simulink model "oog_example"  (R2016a)
settings: Solver=ode5  SolverMode=SingleTasking  StartTime=0.0  StopTime=Ttot  FixedStep=min(Ts_phy,Ts_sim)  RelTol=1e-3
PreLoadFcn:
  | oog_example_init
InitFcn:
  | oog_example_init
values from neighbouring files (symbols this model uses):
  col = {}    [oog_example_init.m]
  flex = {}    [oog_example_init.m]
  systemBase = {}    [oog_example_init.m]
  Ts = Ts_c    (= 0.0001)    [oog_example_init.m]
  Ts_phy = 1*Ts_sim    (= 0.0001)    [oog_example_init.m]
  Ts_sim = 100e-6    (= 0.0001)    [oog_example_init.m]
  wt1 = {}    [oog_example_init.m]
  wt2 = wt1    [oog_example_init.m]
  wt3 = wt1    [oog_example_init.m]
undefined symbols (not defined in the file or in its folder): avr, D1, Delta, DiscIntNeverNeededParam, governor, interface, Lf1, sm
libraries: powerlib x49, simulink_extras x35, pwrsysBasic x30, powerlib_meascontrol x17, pwrsysVICtrl x15, simulink x5, pwrsysVSrc x4, pwrsysTransf x4
(part 2 of 3)

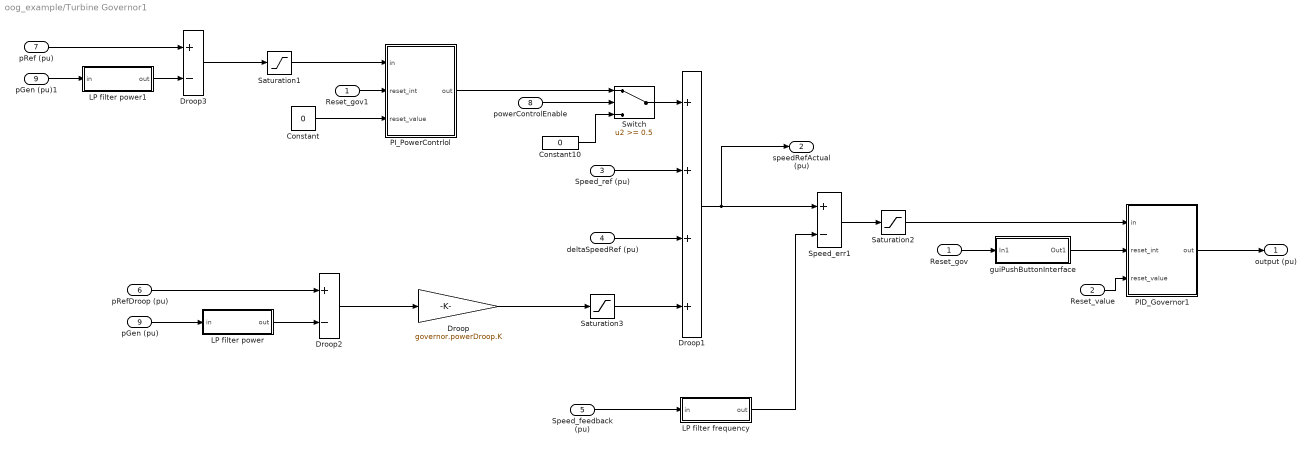
== system oog_example/Turbine Governor1 ==
  Reset_gov : Inport
  Reset_value : Inport  Port=2
  Speed_ref (pu) : Inport  Port=3
  deltaSpeedRef (pu) : Inport  Port=4
  Speed_feedback (pu) : Inport  Port=5
  pRefDroop (pu) : Inport  Port=6
  pRef (pu) : Inport  Port=7
  powerControlEnable : Inport  Port=8
  pGen (pu) : Inport  Port=9
  Constant : Constant  Value=0
  Constant10 : Constant  Value=0  SampleTime=Ts
  Droop : Gain  Gain=governor.powerDroop.K
  Droop1 : Sum  Inputs=++++
  Droop2 : Sum  Inputs=+-
  Droop3 : Sum  Inputs=+-
  LP filter frequency : Subsystem  mask(Discrete first order low pass filter){tau=governor.LPfilterFrequencyMeasurement.T, Ts=Ts, x0=0, y0=0}
      mask prompts: tau "Filter time constant [s]"; Ts "Sampling time [s]"; x0 "Initial input"; y0 "Initial output"
      mask help: Discrete first order low pass filter derived from a continous filter by bilinear transformation.
  LP filter power : Subsystem  mask(Discrete first order low pass filter){tau=governor.LPfilterPowerMeasurementDroop.T, Ts=Ts, x0=0, y0=0}
      mask prompts: tau "Filter time constant [s]"; Ts "Sampling time [s]"; x0 "Initial input"; y0 "Initial output"
      mask help: Discrete first order low pass filter derived from a continous filter by bilinear transformation.
  LP filter power1 : Subsystem  mask(Discrete first order low pass filter){tau=governor.LPfilterPowerMeasurementPowerControl.T, Ts=Ts, x0=0, y0=0}
      mask prompts: tau "Filter time constant [s]"; Ts "Sampling time [s]"; x0 "Initial input"; y0 "Initial output"
      mask help: Discrete first order low pass filter derived from a continous filter by bilinear transformation.
  PID_Governor1 : Subsystem  mask(Discrete PI with parallel form){kp=governor.kP, ki=governor.kI, kd=governor.kd, Tlp=governor.derivativeLP, xi=governor.init, up_sat_limit=governor.saturationUpper, low_sat_limit=governor.saturationLower}
      mask prompts: kp "Proportional gain"; ki "Integral gain"; kd "Derivative gain"; Tlp "Derivative LP filter T"; xi "Initial condition integrator"; up_sat_limit "Saturation upper limit"; low_sat_limit "Saturation lower limit"
      mask help: Discrete PI in parallel form with saturation on the integrator and on the output. The upper and the lower saturation limits are fixed.
  PI_PowerContrlol : Subsystem  mask(Discrete PI with parallel form){kp=governor.powerControl.kP, ki=governor.powerControl.kI, xi=0, up_sat_limit=governor.powerControl.saturationUpper, low_sat_limit=governor.powerControl.saturationLower}
      mask prompts: kp "Proportional gain"; ki "Integral gain"; xi "Initial condition integrator"; up_sat_limit "Saturation upper limit"; low_sat_limit "Saturation lower limit"
      mask help: Discrete PI in parallel form with saturation on the integrator and on the output. The upper and the lower saturation limits are fixed.
  Reset_gov1 : InportShadow
  Saturation1 : Saturate  UpperLimit=governor.powerControl.errMax  LowerLimit=governor.powerControl.errMin
  Saturation2 : Saturate  UpperLimit=governor.speedErrMax  LowerLimit=governor.speedErrMin
  Saturation3 : Saturate  UpperLimit=governor.powerMeasSaturationUpper  LowerLimit=governor.powerMeasSaturationLower
  Speed_err1 : Sum  Inputs=+-
  Switch : Switch  Threshold=0.5
  guiPushButtonInterface : Subsystem
  pGen (pu)1 : InportShadow  Port=9
  output (pu) : Outport
  speedRefActual (pu) : Outport  Port=2
  wires:
  guiPushButtonInterface/1(Out1) -> PID_Governor1/2(reset_int)
  powerControlEnable/1 -> Switch/2
  PI_PowerContrlol/1(out) -> Switch/1
  Constant10/1 -> Switch/3
  Switch/1 -> Droop1/1
  LP filter power1/1(out) -> Droop3/2
  Saturation3/1 -> Droop1/4
  pGen (pu)1/1 -> LP filter power1/1(in)
  Saturation2/1 -> PID_Governor1/1(in)
  deltaSpeedRef (pu)/1 -> Droop1/3
  Constant/1 -> PI_PowerContrlol/3(reset_value)
  Reset_gov1/1 -> PI_PowerContrlol/2(reset_int)
  Saturation1/1 -> PI_PowerContrlol/1(in)
  Droop3/1 -> Saturation1/1
  pRef (pu)/1 -> Droop3/1
  Droop2/1 -> Droop/1
  Reset_value/1 -> PID_Governor1/3(reset_value)
  LP filter power/1(out) -> Droop2/2
  pRefDroop (pu)/1 -> Droop2/1
  pGen (pu)/1 -> LP filter power/1(in)
  Speed_err1/1 -> Saturation2/1
  Droop/1 -> Saturation3/1
  LP filter frequency/1(out) -> Speed_err1/2
  PID_Governor1/1(out) -> output (pu)/1
  Reset_gov/1 -> guiPushButtonInterface/1(In1)
  Droop1/1 -> Speed_err1/1, speedRefActual (pu)/1
  Speed_feedback (pu)/1 -> LP filter frequency/1(in)
  Speed_ref (pu)/1 -> Droop1/2

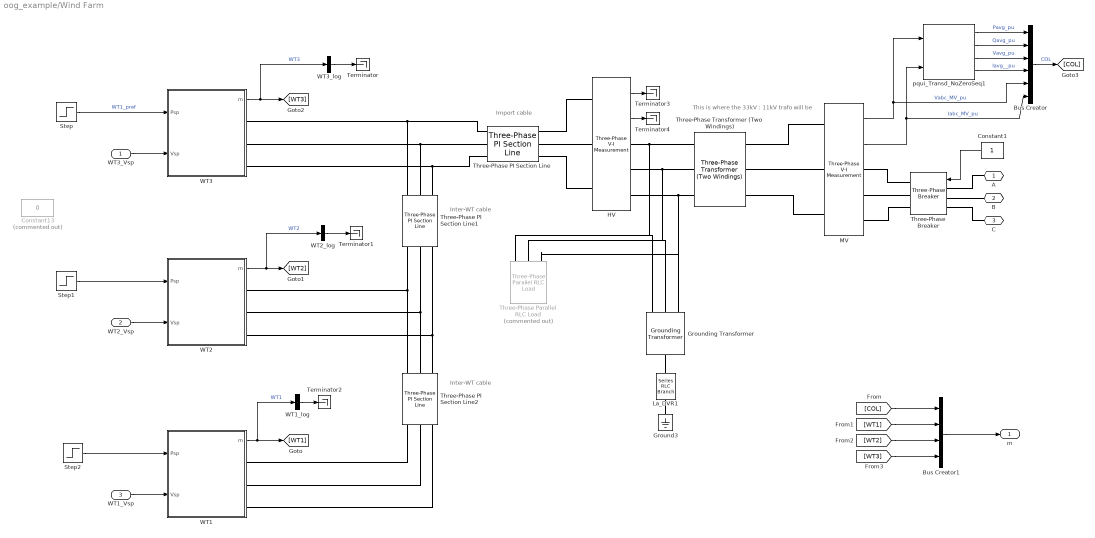
== system oog_example/Wind Farm ==
  note: Import cable
  note: This is where the 33kV : 11kV trafo will be
  note: Inter-WT cable
  note: Inter-WT cable
  WT3_Vsp : Inport
  WT2_Vsp : Inport  Port=2
  WT1_Vsp : Inport  Port=3
  Bus Creator : BusCreator  Inputs=6
  Bus Creator1 : BusCreator  Inputs=4
  Constant1 : Constant  SampleTime=Ts_sim
  Constant13 : Constant  Commented=on  Value=0  SampleTime=Ts_sim
  Ground3 : powerlib/Elements/Ground  LConnTagsString=a
  "Grounding Transformer " : powerlib/Elements/Grounding Transformer   UNITS=pu  NominalPower=[ col.Sn , systemBase.fn ]  NominalVoltage=systemBase.Vn  ZeroSequenceImpedance_pu=[0.025 0.75]  MagnetizationBranch_pu=[500 500]  ZeroSequenceImpedance_SI=[0.052083 589.05]  MagnetizationBranch_SI=[1041.7 3.927e+005]  Measurements=None
  HV : powerlib/Measurements/Three-Phase V-I Measurement  VoltageMeasurement=phase-to-ground  SetLabelV=off  LabelV=vgrid  Vpu=off  VpuLL=off  CurrentMeasurement=yes  SetLabelI=off  LabelI=igrid  Ipu=off  Pbase=sn  Vbase=uab  OutputType=Complex  PhasorSimulation=off  PSBequivalent=0
  La_DVR1 : powerlib/Elements/Series RLC Branch  LConnTagsString=__new0  RConnTagsString=__new0  BranchType=R  Resistance=250  Inductance=Lf1  SetiL0=off  InitialCurrent=0  Capacitance=1.0  Setx0=off  InitialVoltage=0  Measurements=None
  MV : powerlib/Measurements/Three-Phase V-I Measurement  VoltageMeasurement=phase-to-ground  SetLabelV=off  LabelV=vgrid  Vpu=off  VpuLL=off  CurrentMeasurement=yes  SetLabelI=off  LabelI=igrid  Ipu=off  Pbase=sn  Vbase=uab  OutputType=Complex  PhasorSimulation=off  PSBequivalent=0
  Step : Step  Time=6  After=0.73  SampleTime=0
  Step1 : Step  Time=5  After=0.72  SampleTime=0
  Step2 : Step  Time=4  After=0.71  SampleTime=0
  Terminator{,1..4} (5 alike) : Terminator
  Three-Phase PI Section Line : powerlib/Elements/Three-Phase PI Section Line  LConnTagsString=a|b|c  RConnTagsString=A|B|C  Frequency=systemBase.fn  Resistances=[ col.Cable.Rpos col.Cable.Rzero]  Inductances=[ col.Cable.Lpos col.Cable.Lzero]  Capacitances=[col.Cable.Cpos col.Cable.Czero]  Length=col.Cable.Limport
  Three-Phase PI Section Line1 : powerlib/Elements/Three-Phase PI Section Line  LConnTagsString=a|b|c  RConnTagsString=A|B|C  Frequency=systemBase.fn  Resistances=[ col.Cable.Rpos col.Cable.Rzero]  Inductances=[ col.Cable.Lpos col.Cable.Lzero]  Capacitances=[col.Cable.Cpos col.Cable.Czero]  Length=col.Cable.LinterWT
  Three-Phase PI Section Line2 : powerlib/Elements/Three-Phase PI Section Line  LConnTagsString=a|b|c  RConnTagsString=A|B|C  Frequency=systemBase.fn  Resistances=[ col.Cable.Rpos col.Cable.Rzero]  Inductances=[ col.Cable.Lpos col.Cable.Lzero]  Capacitances=[col.Cable.Cpos col.Cable.Czero]  Length=col.Cable.LinterWT
  Three-Phase Parallel RLC Load : powerlib/Elements/Three-Phase Parallel RLC Load  Commented=on  LConnTagsString=A|B|C  Configuration=Y (grounded)  NominalVoltage=col.Un  Vabc=[1e3 1e3 1e3]  Vabcp=[1e3 1e3 1e3]  NominalFrequency=systemBase.fn  UnbalancedPower=off  ActivePower=100  InductivePower=0  CapacitivePower=0  Pabc=[10e3 9e3 11e3]  QLabc=[100 90 110]  QCabc=[100 90 110]  Pabcp=[10e3 9e3 11e3]  QLabcp=[100 90 110]  QCabcp=[100 90 110]  Measurements=None  LoadType=constant Z
  Three-Phase Transformer (Two Windings) : powerlib/Elements/Three-Phase Transformer (Two Windings)  Winding1Connection=Y  Winding2Connection=Delta (D1)  CoreType=Three-limb core (core-type)  SetSaturation=off  Hysteresis=off  DataFile='hysteresis'  SetInitialFlux=off  Measurements=None  UNITS=pu  NominalPower=[ col.Sn , systemBase.fn ]  Winding1=[ systemBase.Vn , col.Trafo.rsc/2 , col.Trafo.xsc/2 ]  Winding2=[ col.Un , col.Trafo.rsc/2 , col.Trafo.xsc/2 ]  Rm=500  Lm=500  L0=0.5  Saturation=[ 0,0 ; 0.0024,1.2 ; 1.0,1.52 ]  InitialFluxes=[0 0 0]  MoreParameters=off  BreakLoop=off  DataType=off  TransfoNumber=1
  Three-Phase Breaker : powerlib/Elements/Three-Phase Breaker  InitialState=closed  SwitchA=on  SwitchB=on  SwitchC=on  SwitchTimes="[1/60  5/60]"  External=on  BreakerResistance=0.01  SnubberResistance=1e6  SnubberCapacitance=1e9  Measurements=None
  WT1 : Subsystem
  WT1_log : BusSelector  OutputSignals=Pavg_pu,Qavg_pu,Vavg_pu,Vdc_pu,Idc_pu  OutputAsBus=on
  WT2 : Subsystem
  WT2_log : BusSelector  OutputSignals=Pavg_pu,Qavg_pu,Vavg_pu,Vdc_pu,Idc_pu  OutputAsBus=on
  WT3 : Subsystem
  WT3_log : BusSelector  OutputSignals=Pavg_pu,Qavg_pu,Vavg_pu,Vdc_pu,Idc_pu  OutputAsBus=on
  pqui_Transd_NoZeroSeq1 : pwrsysBasic/pqui_Transd_NoZeroSeq  Sn=col.Sn  Uanp=systemBase.Vn_phase*sqrt(2)  Iap=col.Iap*(col.Un/systemBase.Vn_phase)
  A : PMIOPort  Port=1  Side=Right
  B : PMIOPort  Port=2  Side=Right
  C : PMIOPort  Port=3  Side=Right
  m : Outport
  wires:
  Constant1/1 -> Three-Phase Breaker/1
  MV/1 -> Bus Creator/5, pqui_Transd_NoZeroSeq1/1  "Vabc_MV_pu"
  HV/1 -> Terminator3/1
  HV/2 -> Terminator4/1
  MV/2 -> pqui_Transd_NoZeroSeq1/2, Bus Creator/6  "Iabc_MV_pu"
  pqui_Transd_NoZeroSeq1/1 -> Bus Creator/1  "Pavg_pu"
  pqui_Transd_NoZeroSeq1/4 -> Bus Creator/4  "Iavg__pu"
  pqui_Transd_NoZeroSeq1/2 -> Bus Creator/2  "Qavg_pu"
  pqui_Transd_NoZeroSeq1/3 -> Bus Creator/3  "Vavg_pu"
  Bus Creator/1 -> [COL]  "COL"
  WT3/1(m) -> WT3_log/1, [WT3]  "WT3"
  WT2/1(m) -> WT2_log/1, [WT2]  "WT2"
  WT3_Vsp/1 -> WT3/2(Vsp)
  WT2_Vsp/1 -> WT2/2(Vsp)
  WT1_Vsp/1 -> WT1/2(Vsp)
  Bus Creator1/1 -> m/1
  [COL] -> Bus Creator1/1
  [WT1] -> Bus Creator1/2
  [WT2] -> Bus Creator1/3
  [WT3] -> Bus Creator1/4
  WT3_log/1 -> Terminator/1
  WT2_log/1 -> Terminator1/1
  WT1/1(m) -> WT1_log/1, [WT1]  "WT1"
  WT1_log/1 -> Terminator2/1
  Step/1 -> WT3/1(Psp)  "WT1_pref"
  Step1/1 -> WT2/1(Psp)
  Step2/1 -> WT1/1(Psp)
  connections:
  Three-Phase Breaker/RConn3 -- MV/RConn3
  Three-Phase Transformer (Two Windings)/LConn3 -- MV/LConn3
  Three-Phase Transformer (Two Windings)/LConn1 -- MV/LConn1
  Three-Phase Transformer (Two Windings)/LConn2 -- MV/LConn2
  MV/RConn1 -- Three-Phase Breaker/RConn1
  Three-Phase PI Section Line/RConn2 -- HV/LConn2
  Three-Phase Breaker/RConn2 -- MV/RConn2
  HV/LConn1 -- Three-Phase PI Section Line/RConn1
  HV/LConn3 -- Three-Phase PI Section Line/RConn3
  Three-Phase Breaker/LConn2 -- B/RConn1
  Three-Phase PI Section Line1/LConn3 -- WT3/RConn3 -- Three-Phase PI Section Line/LConn3
  Three-Phase Breaker/LConn1 -- A/RConn1
  Three-Phase Breaker/LConn3 -- C/RConn1
  Three-Phase PI Section Line1/LConn2 -- WT3/RConn2 -- Three-Phase PI Section Line/LConn2
  Three-Phase PI Section Line/LConn1 -- WT3/RConn1 -- Three-Phase PI Section Line1/LConn1
  Three-Phase PI Section Line2/LConn1 -- WT2/RConn1 -- Three-Phase PI Section Line1/RConn1
  Three-Phase PI Section Line2/LConn2 -- WT2/RConn2 -- Three-Phase PI Section Line1/RConn2
  Three-Phase PI Section Line2/LConn3 -- WT2/RConn3 -- Three-Phase PI Section Line1/RConn3
  WT1/RConn1 -- Three-Phase PI Section Line2/RConn1
  WT1/RConn2 -- Three-Phase PI Section Line2/RConn2
  WT1/RConn3 -- Three-Phase PI Section Line2/RConn3
  HV/RConn1 -- Three-Phase Parallel RLC Load/LConn1 -- "Grounding Transformer "/LConn3 -- Three-Phase Transformer (Two Windings)/RConn1
  HV/RConn2 -- Three-Phase Parallel RLC Load/LConn2 -- "Grounding Transformer "/LConn2 -- Three-Phase Transformer (Two Windings)/RConn2
  HV/RConn3 -- Three-Phase Parallel RLC Load/LConn3 -- "Grounding Transformer "/LConn1 -- Three-Phase Transformer (Two Windings)/RConn3
  La_DVR1/RConn1 -- "Grounding Transformer "/RConn1
  La_DVR1/LConn1 -- Ground3/LConn1

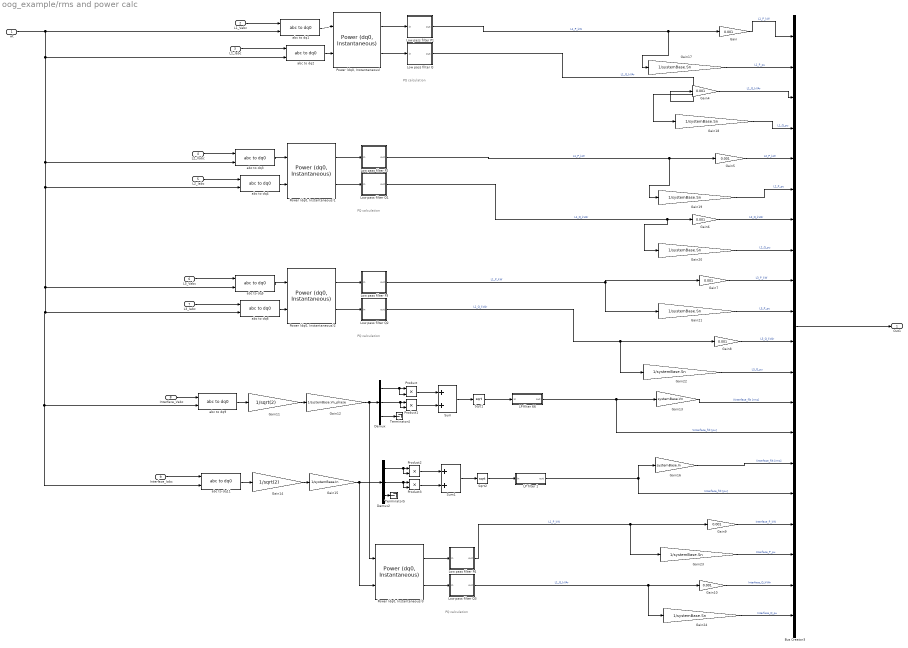
== system oog_example/rms and power calc ==
  note: PQ calculation
  note: PQ calculation
  note: PQ calculation
  note: PQ calculation
  wt : Inport
  L1_Vabc : Inport  Port=2
  L1_Iabc : Inport  Port=3
  L2_Vabc : Inport  Port=4
  L2_Iabc : Inport  Port=5
  L3_Vabc : Inport  Port=6
  L3_Iabc : Inport  Port=7
  Interface_Vabc : Inport  Port=8
  Interface_Iabc : Inport  Port=9
  Bus Creator3 : BusCreator  Inputs=20
  Demux : Demux  Outputs=3
  Demux2 : Demux  Outputs=3
  Gain{,4..10} (8 alike) : Gain  Gain=0.001
  Gain11 : Gain  Gain=1/sqrt(2)
  Gain12 : Gain  Gain=1/systemBase.Vn_phase
  Gain13 : Gain  Gain=systemBase.Vn
  Gain14 : Gain  Gain=1/sqrt(2)
  Gain15 : Gain  Gain=1/systemBase.In
  Gain16 : Gain  Gain=systemBase.In
  Gain{17..24} (8 alike) : Gain  Gain=1/systemBase.Sn
  LP filter 1 : Subsystem  mask(Discrete first order low pass filter){tau=sm.V_measure_T, Ts=Ts, x0=avr.init, y0=avr.init}
      mask prompts: tau "Filter time constant [s]"; Ts "Sampling time [s]"; x0 "Initial input"; y0 "Initial output"
      mask help: Discrete first order low pass filter derived from a continous filter by bilinear transformation.
  LP filter 66 : Subsystem  mask(Discrete first order low pass filter){tau=sm.V_measure_T, Ts=Ts, x0=avr.init, y0=avr.init}
      mask prompts: tau "Filter time constant [s]"; Ts "Sampling time [s]"; x0 "Initial input"; y0 "Initial output"
      mask help: Discrete first order low pass filter derived from a continous filter by bilinear transformation.
  Low pass filter P1 : Subsystem  mask(Discrete first order low pass filter){tau=sm.P_measure, Ts=Ts, x0=0, y0=0}
      mask prompts: tau "Filter time constant [s]"; Ts "Sampling time [s]"; x0 "Initial input"; y0 "Initial output"
      mask help: Discrete first order low pass filter derived from a continous filter by bilinear transformation.
  Low pass filter P2 : Subsystem  mask(Discrete first order low pass filter){tau=sm.P_measure, Ts=Ts, x0=0, y0=0}
      mask prompts: tau "Filter time constant [s]"; Ts "Sampling time [s]"; x0 "Initial input"; y0 "Initial output"
      mask help: Discrete first order low pass filter derived from a continous filter by bilinear transformation.
  Low pass filter P3 : Subsystem  mask(Discrete first order low pass filter){tau=sm.P_measure, Ts=Ts, x0=0, y0=0}
      mask prompts: tau "Filter time constant [s]"; Ts "Sampling time [s]"; x0 "Initial input"; y0 "Initial output"
      mask help: Discrete first order low pass filter derived from a continous filter by bilinear transformation.
  Low pass filter P4 : Subsystem  mask(Discrete first order low pass filter){tau=sm.P_measure, Ts=Ts, x0=0, y0=0}
      mask prompts: tau "Filter time constant [s]"; Ts "Sampling time [s]"; x0 "Initial input"; y0 "Initial output"
      mask help: Discrete first order low pass filter derived from a continous filter by bilinear transformation.
  Low pass filter Q : Subsystem  mask(Discrete first order low pass filter){tau=sm.Q_measure, Ts=Ts, x0=0, y0=0}
      mask prompts: tau "Filter time constant [s]"; Ts "Sampling time [s]"; x0 "Initial input"; y0 "Initial output"
      mask help: Discrete first order low pass filter derived from a continous filter by bilinear transformation.
  Low pass filter Q1 : Subsystem  mask(Discrete first order low pass filter){tau=sm.Q_measure, Ts=Ts, x0=0, y0=0}
      mask prompts: tau "Filter time constant [s]"; Ts "Sampling time [s]"; x0 "Initial input"; y0 "Initial output"
      mask help: Discrete first order low pass filter derived from a continous filter by bilinear transformation.
  Low pass filter Q2 : Subsystem  mask(Discrete first order low pass filter){tau=sm.Q_measure, Ts=Ts, x0=0, y0=0}
      mask prompts: tau "Filter time constant [s]"; Ts "Sampling time [s]"; x0 "Initial input"; y0 "Initial output"
      mask help: Discrete first order low pass filter derived from a continous filter by bilinear transformation.
  Low pass filter Q3 : Subsystem  mask(Discrete first order low pass filter){tau=sm.Q_measure, Ts=Ts, x0=0, y0=0}
      mask prompts: tau "Filter time constant [s]"; Ts "Sampling time [s]"; x0 "Initial input"; y0 "Initial output"
      mask help: Discrete first order low pass filter derived from a continous filter by bilinear transformation.
  Power (dq0, Instantaneous){,1..3} (4 alike) : powerlib_meascontrol/Measurements/Power (dq0, Instantaneous)
  Product{,1..3} (4 alike) : Product
  Sqrt1 : Sqrt  SaturateOnIntegerOverflow=on
  Sqrt2 : Sqrt  SaturateOnIntegerOverflow=on
  Sum : Sum
  Sum1 : Sum
  Terminator4 : Terminator
  Terminator5 : Terminator
  abc to dq{1..6,9,11} (8 alike) : powerlib_meascontrol/Transformations/abc to dq0  Alignment=Aligned with phase A axis
  Out1 : Outport
  wires:
  "Power (dq0, Instantaneous)"/1 -> Low pass filter P1/1(in)
  Gain22/1 -> Bus Creator3/12  "L3_Q_pu"
  Gain24/1 -> Bus Creator3/20  "Interface_Q_pu"
  Gain19/1 -> Bus Creator3/6  "L2_P_pu"
  Gain5/1 -> Bus Creator3/5  "L2_P_kW"
  Gain18/1 -> Bus Creator3/4  "L1_Q_pu"
  Gain4/1 -> Bus Creator3/3  "L1_Q_kVAr"
  Gain17/1 -> Bus Creator3/2  "L1_P_pu"
  wt/1 -> abc to dq1/2, abc to dq2/2, abc to dq3/2, abc to dq4/2, abc to dq5/2, abc to dq9/2, abc to dq11/2, abc to dq6/2
  Interface_Iabc/1 -> abc to dq11/1
  abc to dq11/1 -> Gain14/1
  Gain21/1 -> Bus Creator3/10  "L3_P_pu"
  Sqrt2/1 -> LP filter 1/1(in)
  Gain23/1 -> Bus Creator3/18  "Interface_P_pu"
  Gain20/1 -> Bus Creator3/8  "L2_Q_pu"
  Gain10/1 -> Bus Creator3/19  "Interface_Q_kVAr"
  "Power (dq0, Instantaneous)3"/2 -> Low pass filter Q3/1(in)
  LP filter 1/1(out) -> Gain16/1, Bus Creator3/16  "Iinterface_filt [pu]"
  Interface_Vabc/1 -> abc to dq9/1
  Low pass filter Q2/1(out) -> Gain22/1, Gain8/1  "L1_Q_kVAr"
  "Power (dq0, Instantaneous)3"/1 -> Low pass filter P4/1(in)
  Low pass filter P3/1(out) -> Gain7/1, Gain21/1  "L1_P_kW"
  abc to dq9/1 -> Gain11/1
  Low pass filter P4/1(out) -> Gain9/1, Gain23/1  "L1_P_kW"
  Gain16/1 -> Bus Creator3/15  "Iinterfase_filt [rms]"
  Product2/1 -> Sum1/1
  Demux2/1 -> Product2/1, Product2/2
  LP filter 66/1(out) -> Bus Creator3/14, Gain13/1  "Vinterface_filt [pu]"
  Product/1 -> Sum/1
  Gain11/1 -> Gain12/1
  Gain9/1 -> Bus Creator3/17  "Interface_P_kW"
  Sum/1 -> Sqrt1/1
  Gain15/1 -> Demux2/1, "Power (dq0, Instantaneous)3"/2
  Gain12/1 -> Demux/1, "Power (dq0, Instantaneous)3"/1
  Product3/1 -> Sum1/2
  Product1/1 -> Sum/2
  Demux/1 -> Product/1, Product/2
  Low pass filter Q3/1(out) -> Gain24/1, Gain10/1  "L1_Q_kVAr"
  Sqrt1/1 -> LP filter 66/1(in)
  Gain14/1 -> Gain15/1
  Demux2/2 -> Product3/1, Product3/2
  Gain13/1 -> Bus Creator3/13  "Vinterfase_filt [rms]"
  Sum1/1 -> Sqrt2/1
  Demux/2 -> Product1/1, Product1/2
  "Power (dq0, Instantaneous)1"/1 -> Low pass filter P2/1(in)
  Gain8/1 -> Bus Creator3/11  "L3_Q_kVAr"
  L3_Vabc/1 -> abc to dq5/1
  L2_Iabc/1 -> abc to dq4/1
  L2_Vabc/1 -> abc to dq3/1
  abc to dq3/1 -> "Power (dq0, Instantaneous)1"/1
  Gain7/1 -> Bus Creator3/9  "L3_P_kW"
  L3_Iabc/1 -> abc to dq6/1
  "Power (dq0, Instantaneous)2"/1 -> Low pass filter P3/1(in)
  Low pass filter Q/1(out) -> Gain4/1, Gain18/1  "L1_Q_kVAr"
  "Power (dq0, Instantaneous)1"/2 -> Low pass filter Q1/1(in)
  "Power (dq0, Instantaneous)2"/2 -> Low pass filter Q2/1(in)
  abc to dq4/1 -> "Power (dq0, Instantaneous)1"/2
  Low pass filter P1/1(out) -> Gain/1, Gain17/1  "L1_P_kW"
  abc to dq5/1 -> "Power (dq0, Instantaneous)2"/1
  Low pass filter Q1/1(out) -> Gain6/1, Gain20/1  "L1_Q_kVAr"
  Bus Creator3/1 -> Out1/1
  abc to dq6/1 -> "Power (dq0, Instantaneous)2"/2
  Low pass filter P2/1(out) -> Gain5/1, Gain19/1  "L1_P_kW"
  Gain6/1 -> Bus Creator3/7  "L2_Q_kVAr"
  L1_Iabc/1 -> abc to dq2/1
  L1_Vabc/1 -> abc to dq1/1
  abc to dq2/1 -> "Power (dq0, Instantaneous)"/2
  abc to dq1/1 -> "Power (dq0, Instantaneous)"/1
  Gain/1 -> Bus Creator3/1  "L1_P_kW"
  "Power (dq0, Instantaneous)"/2 -> Low pass filter Q/1(in)
  Demux2/3 -> Terminator5/1
  Demux/3 -> Terminator4/1

== system oog_example/Automatic voltage regulator/LP filter active power ==
  in : Inport
  Discrete Transfer Fcn (with initial outputs) : simulink_extras/Additional Discrete/Discrete Transfer Fcn (with initial outputs)  N=[1/tau*Ts/2 1/tau*Ts/2]  D=[(1/tau*Ts/2+1) (1/tau*Ts/2-1)]  U0=x0  Y0=y0  TS=Ts
  out : Outport
  wires:
  in/1 -> Discrete Transfer Fcn (with initial outputs)/1
  Discrete Transfer Fcn (with initial outputs)/1 -> out/1

== system oog_example/Automatic voltage regulator/LP filter frequency ==
  in : Inport
  Discrete Transfer Fcn (with initial outputs) : simulink_extras/Additional Discrete/Discrete Transfer Fcn (with initial outputs)  N=[1/tau*Ts/2 1/tau*Ts/2]  D=[(1/tau*Ts/2+1) (1/tau*Ts/2-1)]  U0=x0  Y0=y0  TS=Ts
  out : Outport
  wires:
  Discrete Transfer Fcn (with initial outputs)/1 -> out/1
  in/1 -> Discrete Transfer Fcn (with initial outputs)/1

== system oog_example/Automatic voltage regulator/LP filter frequency1 ==
  in : Inport
  Discrete Transfer Fcn (with initial outputs) : simulink_extras/Additional Discrete/Discrete Transfer Fcn (with initial outputs)  N=[1/tau*Ts/2 1/tau*Ts/2]  D=[(1/tau*Ts/2+1) (1/tau*Ts/2-1)]  U0=x0  Y0=y0  TS=Ts
  out : Outport
  wires:
  Discrete Transfer Fcn (with initial outputs)/1 -> out/1
  in/1 -> Discrete Transfer Fcn (with initial outputs)/1

== system oog_example/Automatic voltage regulator/LP filter reactive power ==
  in : Inport
  Discrete Transfer Fcn (with initial outputs) : simulink_extras/Additional Discrete/Discrete Transfer Fcn (with initial outputs)  N=[1/tau*Ts/2 1/tau*Ts/2]  D=[(1/tau*Ts/2+1) (1/tau*Ts/2-1)]  U0=x0  Y0=y0  TS=Ts
  out : Outport
  wires:
  Discrete Transfer Fcn (with initial outputs)/1 -> out/1
  in/1 -> Discrete Transfer Fcn (with initial outputs)/1

== system oog_example/Automatic voltage regulator/PID_Governor1 ==
  in : Inport
  reset_int : Inport  Port=2
  reset_value : Inport  Port=3
  Discrete Derivative : simulink/Discrete/Discrete Derivative  gainval=1.0  ICPrevScaledInput=0.0  InputProcessing=Inherited  OutMin=[]  OutMax=[]  OutDataType=fixdt(1, 16)  OutScaling=2^-10  DoSatur=off
  Discrete-Time Integrator : DiscreteIntegrator  IntegratorMethod=Integration: Trapezoidal  ExternalReset=level  InitialConditionSource=external  InitialCondition=xi  InitialConditionSetting=State (most efficient)  SampleTime=Ts  LimitOutput=on  UpperSaturationLimit=up_sat_limit  LowerSaturationLimit=low_sat_limit  ICPrevOutput=DiscIntNeverNeededParam  ICPrevScaledInput=DiscIntNeverNeededParam
  Integral Gain : Gain  DisableCoverage=on  Gain=ki
  Integral Gain1 : Gain  DisableCoverage=on  Gain=kd
  LP filter power : Subsystem  mask(Discrete first order low pass filter){tau=governor.derivativeLP, Ts=Ts, x0=0, y0=0}
      mask prompts: tau "Filter time constant [s]"; Ts "Sampling time [s]"; x0 "Initial input"; y0 "Initial output"
      mask help: Discrete first order low pass filter derived from a continous filter by bilinear transformation.
  P+I : Sum  Inputs=+++
  Proportional Gain : Gain  DisableCoverage=on  Gain=kp
  Saturation : Saturate  UpperLimit=up_sat_limit  LowerLimit=low_sat_limit
  out : Outport
  wires:
  LP filter power/1(out) -> Discrete Derivative/1
  Discrete Derivative/1 -> P+I/3
  Integral Gain1/1 -> LP filter power/1(in)
  reset_value/1 -> Discrete-Time Integrator/3
  reset_int/1 -> Discrete-Time Integrator/2
  Saturation/1 -> out/1
  Proportional Gain/1 -> P+I/1
  in/1 -> Integral Gain/1, Integral Gain1/1, Proportional Gain/1
  P+I/1 -> Saturation/1
  Integral Gain/1 -> Discrete-Time Integrator/1
  Discrete-Time Integrator/1 -> P+I/2

== system oog_example/Automatic voltage regulator/guiPushButtonInterface ==
  In1 : Inport
  Data Type Conversion6 : DataTypeConversion  OutDataTypeStr=double  RndMeth=Round
  Detect Change : simulink/Logic and Bit Operations/Detect Change  vinit=0  InputProcessing=Inherited  OutDataTypeStr=boolean
  IC1 : InitialCondition  Value=0
  Out1 : Outport
  wires:
  IC1/1 -> Out1/1
  Data Type Conversion6/1 -> IC1/1
  Detect Change/1 -> Data Type Conversion6/1
  In1/1 -> Detect Change/1

== system oog_example/Rotation1/guiPushButtonInterface ==
  In1 : Inport
  Data Type Conversion6 : DataTypeConversion  OutDataTypeStr=double  RndMeth=Round
  Detect Change : simulink/Logic and Bit Operations/Detect Change  vinit=0  InputProcessing=Inherited  OutDataTypeStr=boolean
  IC1 : InitialCondition  Value=0
  Out1 : Outport
  wires:
  IC1/1 -> Out1/1
  Data Type Conversion6/1 -> IC1/1
  Detect Change/1 -> Data Type Conversion6/1
  In1/1 -> Detect Change/1

== system oog_example/SM_simple/LP filter  ==
  in : Inport
  Discrete Transfer Fcn (with initial outputs) : simulink_extras/Additional Discrete/Discrete Transfer Fcn (with initial outputs)  N=[1/tau*Ts/2 1/tau*Ts/2]  D=[(1/tau*Ts/2+1) (1/tau*Ts/2-1)]  U0=x0  Y0=y0  TS=Ts
  out : Outport
  wires:
  Discrete Transfer Fcn (with initial outputs)/1 -> out/1
  in/1 -> Discrete Transfer Fcn (with initial outputs)/1

== system oog_example/SM_simple/LP filter 1 ==
  in : Inport
  Discrete Transfer Fcn (with initial outputs) : simulink_extras/Additional Discrete/Discrete Transfer Fcn (with initial outputs)  N=[1/tau*Ts/2 1/tau*Ts/2]  D=[(1/tau*Ts/2+1) (1/tau*Ts/2-1)]  U0=x0  Y0=y0  TS=Ts
  out : Outport
  wires:
  Discrete Transfer Fcn (with initial outputs)/1 -> out/1
  in/1 -> Discrete Transfer Fcn (with initial outputs)/1

== system oog_example/SM_simple/LP filter 2 ==
  in : Inport
  Discrete Transfer Fcn (with initial outputs) : simulink_extras/Additional Discrete/Discrete Transfer Fcn (with initial outputs)  N=[1/tau*Ts/2 1/tau*Ts/2]  D=[(1/tau*Ts/2+1) (1/tau*Ts/2-1)]  U0=x0  Y0=y0  TS=Ts
  out : Outport
  wires:
  in/1 -> Discrete Transfer Fcn (with initial outputs)/1
  Discrete Transfer Fcn (with initial outputs)/1 -> out/1

== system oog_example/SM_simple/LP filter 3 ==
  in : Inport
  Discrete Transfer Fcn (with initial outputs) : simulink_extras/Additional Discrete/Discrete Transfer Fcn (with initial outputs)  N=[1/tau*Ts/2 1/tau*Ts/2]  D=[(1/tau*Ts/2+1) (1/tau*Ts/2-1)]  U0=x0  Y0=y0  TS=Ts
  out : Outport
  wires:
  in/1 -> Discrete Transfer Fcn (with initial outputs)/1
  Discrete Transfer Fcn (with initial outputs)/1 -> out/1

== system oog_example/SM_simple/LP filter 3  ==
  in : Inport
  Discrete Transfer Fcn (with initial outputs) : simulink_extras/Additional Discrete/Discrete Transfer Fcn (with initial outputs)  N=[1/tau*Ts/2 1/tau*Ts/2]  D=[(1/tau*Ts/2+1) (1/tau*Ts/2-1)]  U0=x0  Y0=y0  TS=Ts
  out : Outport
  wires:
  Discrete Transfer Fcn (with initial outputs)/1 -> out/1
  in/1 -> Discrete Transfer Fcn (with initial outputs)/1

== system oog_example/SM_simple/LP filter 3 1 ==
  in : Inport
  Discrete Transfer Fcn (with initial outputs) : simulink_extras/Additional Discrete/Discrete Transfer Fcn (with initial outputs)  N=[1/tau*Ts/2 1/tau*Ts/2]  D=[(1/tau*Ts/2+1) (1/tau*Ts/2-1)]  U0=x0  Y0=y0  TS=Ts
  out : Outport
  wires:
  Discrete Transfer Fcn (with initial outputs)/1 -> out/1
  in/1 -> Discrete Transfer Fcn (with initial outputs)/1

== system oog_example/SM_simple/LP filter 3 2 ==
  in : Inport
  Discrete Transfer Fcn (with initial outputs) : simulink_extras/Additional Discrete/Discrete Transfer Fcn (with initial outputs)  N=[1/tau*Ts/2 1/tau*Ts/2]  D=[(1/tau*Ts/2+1) (1/tau*Ts/2-1)]  U0=x0  Y0=y0  TS=Ts
  out : Outport
  wires:
  Discrete Transfer Fcn (with initial outputs)/1 -> out/1
  in/1 -> Discrete Transfer Fcn (with initial outputs)/1

== system oog_example/SM_simple/LP filter 4 ==
  in : Inport
  Discrete Transfer Fcn (with initial outputs) : simulink_extras/Additional Discrete/Discrete Transfer Fcn (with initial outputs)  N=[1/tau*Ts/2 1/tau*Ts/2]  D=[(1/tau*Ts/2+1) (1/tau*Ts/2-1)]  U0=x0  Y0=y0  TS=Ts
  out : Outport
  wires:
  Discrete Transfer Fcn (with initial outputs)/1 -> out/1
  in/1 -> Discrete Transfer Fcn (with initial outputs)/1

== system oog_example/SM_simple/LP filter 5 ==
  in : Inport
  Discrete Transfer Fcn (with initial outputs) : simulink_extras/Additional Discrete/Discrete Transfer Fcn (with initial outputs)  N=[1/tau*Ts/2 1/tau*Ts/2]  D=[(1/tau*Ts/2+1) (1/tau*Ts/2-1)]  U0=x0  Y0=y0  TS=Ts
  out : Outport
  wires:
  Discrete Transfer Fcn (with initial outputs)/1 -> out/1
  in/1 -> Discrete Transfer Fcn (with initial outputs)/1

== system oog_example/SM_simple/LP filter 6 ==
  in : Inport
  Discrete Transfer Fcn (with initial outputs) : simulink_extras/Additional Discrete/Discrete Transfer Fcn (with initial outputs)  N=[1/tau*Ts/2 1/tau*Ts/2]  D=[(1/tau*Ts/2+1) (1/tau*Ts/2-1)]  U0=x0  Y0=y0  TS=Ts
  out : Outport
  wires:
  in/1 -> Discrete Transfer Fcn (with initial outputs)/1
  Discrete Transfer Fcn (with initial outputs)/1 -> out/1

== system oog_example/SM_simple/LP filter 66 ==
  in : Inport
  Discrete Transfer Fcn (with initial outputs) : simulink_extras/Additional Discrete/Discrete Transfer Fcn (with initial outputs)  N=[1/tau*Ts/2 1/tau*Ts/2]  D=[(1/tau*Ts/2+1) (1/tau*Ts/2-1)]  U0=x0  Y0=y0  TS=Ts
  out : Outport
  wires:
  Discrete Transfer Fcn (with initial outputs)/1 -> out/1
  in/1 -> Discrete Transfer Fcn (with initial outputs)/1

== system oog_example/SM_simple/LP filter 67 ==
  in : Inport
  Discrete Transfer Fcn (with initial outputs) : simulink_extras/Additional Discrete/Discrete Transfer Fcn (with initial outputs)  N=[1/tau*Ts/2 1/tau*Ts/2]  D=[(1/tau*Ts/2+1) (1/tau*Ts/2-1)]  U0=x0  Y0=y0  TS=Ts
  out : Outport
  wires:
  Discrete Transfer Fcn (with initial outputs)/1 -> out/1
  in/1 -> Discrete Transfer Fcn (with initial outputs)/1

== system oog_example/SM_simple/Low pass filter P1 ==
  in : Inport
  Discrete Transfer Fcn (with initial outputs) : simulink_extras/Additional Discrete/Discrete Transfer Fcn (with initial outputs)  N=[1/tau*Ts/2 1/tau*Ts/2]  D=[(1/tau*Ts/2+1) (1/tau*Ts/2-1)]  U0=x0  Y0=y0  TS=Ts
  out : Outport
  wires:
  Discrete Transfer Fcn (with initial outputs)/1 -> out/1
  in/1 -> Discrete Transfer Fcn (with initial outputs)/1

== system oog_example/SM_simple/Low pass filter Q ==
  in : Inport
  Discrete Transfer Fcn (with initial outputs) : simulink_extras/Additional Discrete/Discrete Transfer Fcn (with initial outputs)  N=[1/tau*Ts/2 1/tau*Ts/2]  D=[(1/tau*Ts/2+1) (1/tau*Ts/2-1)]  U0=x0  Y0=y0  TS=Ts
  out : Outport
  wires:
  Discrete Transfer Fcn (with initial outputs)/1 -> out/1
  in/1 -> Discrete Transfer Fcn (with initial outputs)/1

== system oog_example/SM_simple/powerCalcAndFilt1 ==
  note: Low pass filter power measurement
  Vabc : Inport
  Iabc : Inport  Port=2
  LP filter frequency1 : Subsystem  mask(Discrete first order low pass filter){tau=sm.P_measure, Ts=Ts, x0=avr.init, y0=avr.init}
      mask prompts: tau "Filter time constant [s]"; Ts "Sampling time [s]"; x0 "Initial input"; y0 "Initial output"
      mask help: Discrete first order low pass filter derived from a continous filter by bilinear transformation.
  LP filter frequency2 : Subsystem  mask(Discrete first order low pass filter){tau=sm.Q_measure, Ts=Ts, x0=avr.init, y0=avr.init}
      mask prompts: tau "Filter time constant [s]"; Ts "Sampling time [s]"; x0 "Initial input"; y0 "Initial output"
      mask help: Discrete first order low pass filter derived from a continous filter by bilinear transformation.
  "Power (3ph, Instantaneous)1" : powerlib_meascontrol/Measurements/Power (3ph, Instantaneous)
  P_filt : Outport
  Q_filt1 : Outport  Port=2
  wires:
  LP filter frequency2/1(out) -> Q_filt1/1
  LP filter frequency1/1(out) -> P_filt/1
  "Power (3ph, Instantaneous)1"/2 -> LP filter frequency2/1(in)
  Iabc/1 -> "Power (3ph, Instantaneous)1"/2
  Vabc/1 -> "Power (3ph, Instantaneous)1"/1
  "Power (3ph, Instantaneous)1"/1 -> LP filter frequency1/1(in)

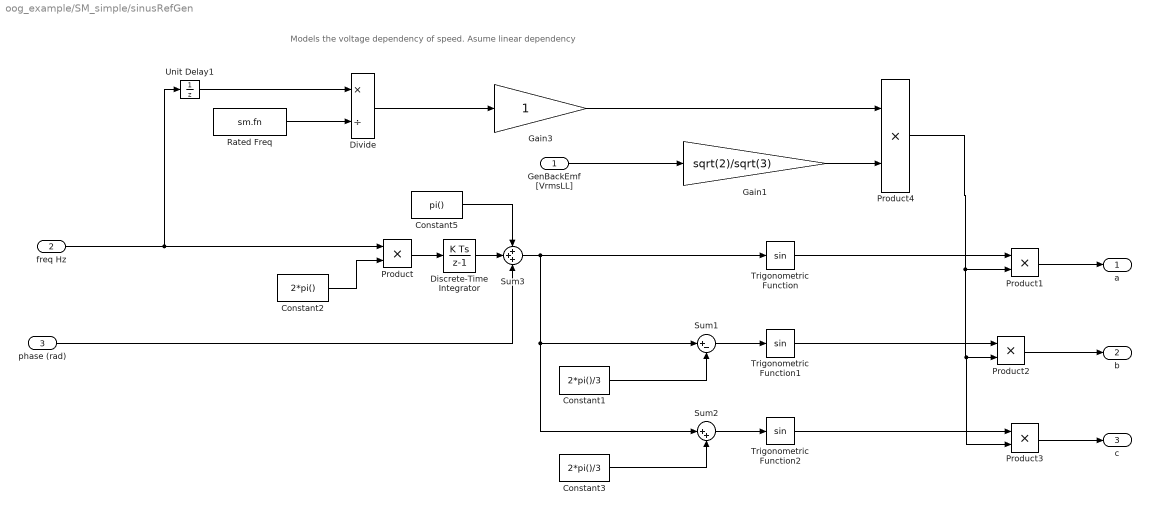
== system oog_example/SM_simple/sinusRefGen ==
  note: Models the voltage dependency of speed. Asume linear dependency
  GenBackEmf [VrmsLL] : Inport
  freq Hz : Inport  Port=2
  phase (rad) : Inport  Port=3
  Constant1 : Constant  Value=2*pi()/3  SampleTime=-1
  Constant2 : Constant  Value=2*pi()  SampleTime=-1
  Constant3 : Constant  Value=2*pi()/3  SampleTime=-1
  Constant5 : Constant  Value=pi()  SampleTime=-1
  Discrete-Time Integrator : DiscreteIntegrator  InitialConditionSetting=State (most efficient)  SampleTime=-1  ICPrevOutput=DiscIntNeverNeededParam  ICPrevScaledInput=DiscIntNeverNeededParam
  Divide : Product  Inputs=*/
  Gain1 : Gain  Gain=sqrt(2)/sqrt(3)
  Gain3 : Gain
  Product{,1..4} (5 alike) : Product
  Rated Freq : Constant  Value=sm.fn  SampleTime=-1
  Sum1 : Sum  Inputs=|+-
  Sum2 : Sum  Inputs=|++
  Sum3 : Sum  Inputs=+++
  Trigonometric Function : Trigonometry
  Trigonometric Function1 : Trigonometry
  Trigonometric Function2 : Trigonometry
  Unit Delay1 : UnitDelay  InitialCondition=sm.fn  SampleTime=-1
  a : Outport
  b : Outport  Port=2
  c : Outport  Port=3
  wires:
  Constant5/1 -> Sum3/1
  Gain3/1 -> Product4/1
  Product4/1 -> Product1/2, Product2/2, Product3/2
  Trigonometric Function2/1 -> Product3/1
  Discrete-Time Integrator/1 -> Sum3/2
  Divide/1 -> Gain3/1
  Rated Freq/1 -> Divide/2
  Constant2/1 -> Product/2
  Trigonometric Function1/1 -> Product2/1
  Product1/1 -> a/1
  Product3/1 -> c/1
  Gain1/1 -> Product4/2
  Product2/1 -> b/1
  GenBackEmf [VrmsLL]/1 -> Gain1/1
  Constant3/1 -> Sum2/2
  Constant1/1 -> Sum1/2
  Sum2/1 -> Trigonometric Function2/1
  Sum1/1 -> Trigonometric Function1/1
  Trigonometric Function/1 -> Product1/1
  Sum3/1 -> Sum2/1, Sum1/1, Trigonometric Function/1
  phase (rad)/1 -> Sum3/3
  Product/1 -> Discrete-Time Integrator/1
  freq Hz/1 -> Product/1, Unit Delay1/1
  Unit Delay1/1 -> Divide/1

== system oog_example/Turbine Governor1/LP filter frequency ==
  in : Inport
  Discrete Transfer Fcn (with initial outputs) : simulink_extras/Additional Discrete/Discrete Transfer Fcn (with initial outputs)  N=[1/tau*Ts/2 1/tau*Ts/2]  D=[(1/tau*Ts/2+1) (1/tau*Ts/2-1)]  U0=x0  Y0=y0  TS=Ts
  out : Outport
  wires:
  Discrete Transfer Fcn (with initial outputs)/1 -> out/1
  in/1 -> Discrete Transfer Fcn (with initial outputs)/1

== system oog_example/Turbine Governor1/LP filter power ==
  in : Inport
  Discrete Transfer Fcn (with initial outputs) : simulink_extras/Additional Discrete/Discrete Transfer Fcn (with initial outputs)  N=[1/tau*Ts/2 1/tau*Ts/2]  D=[(1/tau*Ts/2+1) (1/tau*Ts/2-1)]  U0=x0  Y0=y0  TS=Ts
  out : Outport
  wires:
  Discrete Transfer Fcn (with initial outputs)/1 -> out/1
  in/1 -> Discrete Transfer Fcn (with initial outputs)/1

== system oog_example/Turbine Governor1/LP filter power1 ==
  in : Inport
  Discrete Transfer Fcn (with initial outputs) : simulink_extras/Additional Discrete/Discrete Transfer Fcn (with initial outputs)  N=[1/tau*Ts/2 1/tau*Ts/2]  D=[(1/tau*Ts/2+1) (1/tau*Ts/2-1)]  U0=x0  Y0=y0  TS=Ts
  out : Outport
  wires:
  Discrete Transfer Fcn (with initial outputs)/1 -> out/1
  in/1 -> Discrete Transfer Fcn (with initial outputs)/1

== system oog_example/Turbine Governor1/PID_Governor1 ==
  in : Inport
  reset_int : Inport  Port=2
  reset_value : Inport  Port=3
  Discrete Derivative : simulink/Discrete/Discrete Derivative  gainval=1.0  ICPrevScaledInput=0.0  InputProcessing=Inherited  OutMin=[]  OutMax=[]  OutDataType=fixdt(1, 16)  OutScaling=2^-10  DoSatur=off
  Discrete-Time Integrator : DiscreteIntegrator  IntegratorMethod=Integration: Trapezoidal  ExternalReset=level  InitialConditionSource=external  InitialCondition=xi  InitialConditionSetting=State (most efficient)  SampleTime=Ts  LimitOutput=on  UpperSaturationLimit=up_sat_limit  LowerSaturationLimit=low_sat_limit  ICPrevOutput=DiscIntNeverNeededParam  ICPrevScaledInput=DiscIntNeverNeededParam
  Integral Gain : Gain  DisableCoverage=on  Gain=ki
  Integral Gain1 : Gain  DisableCoverage=on  Gain=kd
  LP filter power : Subsystem  mask(Discrete first order low pass filter){tau=governor.derivativeLP, Ts=Ts, x0=0, y0=0}
      mask prompts: tau "Filter time constant [s]"; Ts "Sampling time [s]"; x0 "Initial input"; y0 "Initial output"
      mask help: Discrete first order low pass filter derived from a continous filter by bilinear transformation.
  P+I : Sum  Inputs=+++
  Proportional Gain : Gain  DisableCoverage=on  Gain=kp
  Saturation : Saturate  UpperLimit=up_sat_limit  LowerLimit=low_sat_limit
  out : Outport
  wires:
  LP filter power/1(out) -> Discrete Derivative/1
  Discrete Derivative/1 -> P+I/3
  Integral Gain1/1 -> LP filter power/1(in)
  reset_value/1 -> Discrete-Time Integrator/3
  reset_int/1 -> Discrete-Time Integrator/2
  Saturation/1 -> out/1
  Proportional Gain/1 -> P+I/1
  in/1 -> Integral Gain/1, Integral Gain1/1, Proportional Gain/1
  P+I/1 -> Saturation/1
  Integral Gain/1 -> Discrete-Time Integrator/1
  Discrete-Time Integrator/1 -> P+I/2

== system oog_example/Turbine Governor1/PI_PowerContrlol ==
  in : Inport
  reset_int : Inport  Port=2
  reset_value : Inport  Port=3
  Discrete-Time Integrator : DiscreteIntegrator  IntegratorMethod=Integration: Trapezoidal  ExternalReset=level  InitialConditionSource=external  InitialCondition=xi  InitialConditionSetting=State (most efficient)  SampleTime=Ts  LimitOutput=on  UpperSaturationLimit=up_sat_limit  LowerSaturationLimit=low_sat_limit  ICPrevOutput=DiscIntNeverNeededParam  ICPrevScaledInput=DiscIntNeverNeededParam
  Integral Gain : Gain  DisableCoverage=on  Gain=ki
  P+I : Sum
  Proportional Gain : Gain  DisableCoverage=on  Gain=kp
  Saturation : Saturate  UpperLimit=up_sat_limit  LowerLimit=low_sat_limit
  out : Outport
  wires:
  reset_value/1 -> Discrete-Time Integrator/3
  reset_int/1 -> Discrete-Time Integrator/2
  Saturation/1 -> out/1
  Proportional Gain/1 -> P+I/1
  in/1 -> Integral Gain/1, Proportional Gain/1
  P+I/1 -> Saturation/1
  Integral Gain/1 -> Discrete-Time Integrator/1
  Discrete-Time Integrator/1 -> P+I/2

== system oog_example/Turbine Governor1/guiPushButtonInterface ==
  In1 : Inport
  Data Type Conversion6 : DataTypeConversion  OutDataTypeStr=double  RndMeth=Round
  Detect Change : simulink/Logic and Bit Operations/Detect Change  vinit=0  InputProcessing=Inherited  OutDataTypeStr=boolean
  IC1 : InitialCondition  Value=0
  Out1 : Outport
  wires:
  IC1/1 -> Out1/1
  Data Type Conversion6/1 -> IC1/1
  Detect Change/1 -> Data Type Conversion6/1
  In1/1 -> Detect Change/1

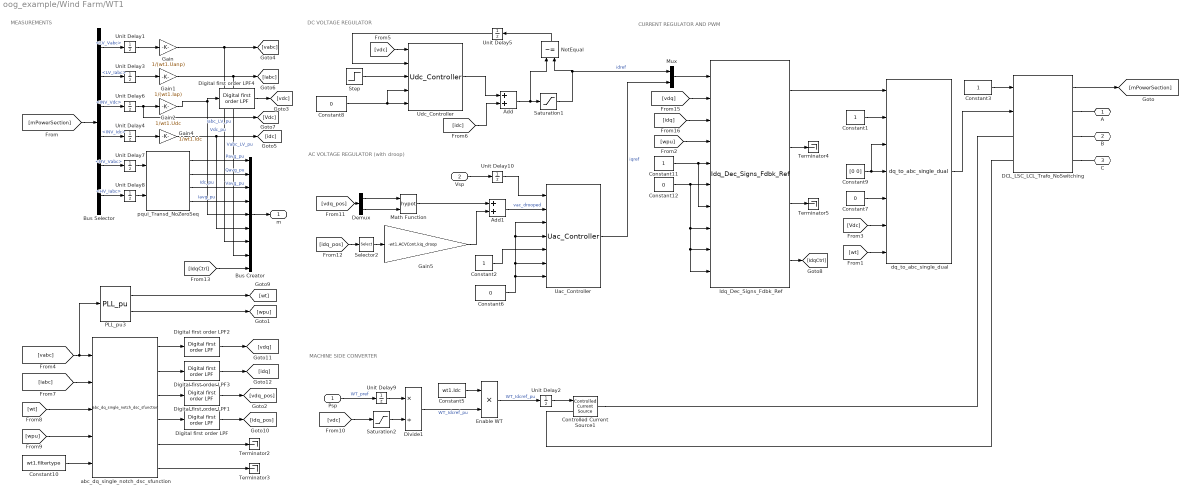
== system oog_example/Wind Farm/WT1 ==
  note: MEASUREMENTS
  note: MACHINE SIDE CONVERTER
  note: AC VOLTAGE REGULATOR (with droop)
  note: DC VOLTAGE REGULATOR
  note: CURRENT REGULATOR AND PWM
  Psp : Inport
  Vsp : Inport  Port=2
  Add : Sum
  Add1 : Sum
  Bus Creator : BusCreator  Inputs=9
  Bus Selector : BusSelector  OutputSignals=LV_Vabc,LV_Iabc,INV_Vdc,INV_Idc,HV_Vabc,HV_Iabc
  Constant1 : Constant  SampleTime=wt1.Ts_control
  Constant10 : Constant  Value=wt1.filtertype  SampleTime=wt1.Ts_control
  Constant11 : Constant  SampleTime=wt2.Ts_control
  Constant12 : Constant  Value=0  SampleTime=wt2.Ts_control
  Constant2 : Constant  SampleTime=wt1.Ts_control
  Constant3 : Constant  SampleTime=wt1.Ts_control
  Constant5 : Constant  Value=wt1.Idc  SampleTime=wt1.Ts_control
  Constant6 : Constant  Value=0  SampleTime=wt1.Ts_control
  Constant7 : Constant  Value=0  SampleTime=wt1.Ts_control
  Constant8 : Constant  Value=0  SampleTime=wt1.Ts_control
  Constant9 : Constant  Value=[0 0]  SampleTime=wt1.Ts_control
  Controlled Current Source1 : powerlib/Electrical Sources/Controlled Current Source  Initialize=on  Source_Type=DC  Amplitude=0  Phase=0  Frequency=50  Measurements=None
  DCL_LSC_LCL_Trafo_NoSwitching : pwrsysVSrc/DCL_LSC_LCL_Trafo_NoSwitching  Sn=wt1.Sn  fn=systemBase.fn  Uhv_ab=col.Un  Uab=wt1.Un  lf2=wt1.LCL.l2  rf2=wt1.LCL.r2  Lf1=wt1.LCL.L1  Rf1=wt1.LCL.R1  Cf=wt1.LCL.Cf  Rc=wt1.LCL.Rf  Cdc=wt1.Cdc  Udc0=wt1.Udc  Tsm=wt1.Ts_control  Tstart=wt1.DCVCont.Start
  Demux : Demux  Outputs=2
  Digital first order LPF{,1..4} (5 alike) : pwrsysBasic/Digital first order LPF  Ts=wt1.Ts_control  fcutout=wt1.CurrCont.f_LPF_noise
  Divide1 : Product  Inputs=*/
  Enable WT : Product  Inputs=**
  Gain : Gain  Gain=1/(wt1.Uanp)
  Gain1 : Gain  Gain=1/(wt1.Iap)
  Gain2 : Gain  Gain=1/wt1.Udc
  Gain4 : Gain  Gain=1/wt1.Idc
  Gain5 : Gain  Gain=-wt1.ACVCont.kiq_droop
  Idq_Dec_Signs_Fdbk_Ref : pwrsysVICtrl/Idq_Dec_Signs_Fdbk_Ref  Ts=wt1.Ts_control  fn=systemBase.fn  Kp=wt1.CurrContSingle.kp  Ti=wt1.CurrContSingle.Ti  L=wt1.CurrCont.x  PI_max=wt1.CurrCont.PImax  PI_min=wt1.CurrCont.PImin  TrafoPhaseComp=0
  Math Function : Math  Operator=hypot  SaturateOnIntegerOverflow=on
  Mux : Mux  Inputs=2
  NotEqual : RelationalOperator  Operator=~=  OutDataTypeStr=boolean
  PLL_pu3 : pwrsysBasic/PLL_pu  fn=systemBase.fn  Ts=wt1.Ts_control  Kp_pll=90  Ki_pll=1200  Kd_pll=0  PLL_ini=60
  Saturation1 : Saturate  UpperLimit=wt1.DCVCont.PImax  LowerLimit=wt1.DCVCont.PImin
  Saturation2 : Saturate  UpperLimit=1.2  LowerLimit=0.8
  Selector2 : Selector  IndexMode=Zero-based  InputPortWidth=2  IndexOptions=Index vector (dialog)  Indices=1  OutputSizes=1
  Step : Step  Time=wt1.DCVCont.Start  SampleTime=0
  Terminator{2..5} (4 alike) : Terminator
  Uac_Controller : pwrsysVICtrl/Uac_Controller  Ts=wt1.Ts_control  Kg=wt1.ACVCont.kg  Kp=wt1.ACVCont.kp  Ti=wt1.ACVCont.Ti  PI_max=wt1.ACVCont.PImax  PI_min=wt1.ACVCont.PImin
  Udc_Controller : pwrsysVICtrl/Udc_Controller  Ts=wt1.Ts_control  Kp=wt1.DCVContSingle.kp  Ti=wt1.DCVContSingle.Ti  PI_max=wt1.DCVCont.PImax  PI_min=wt1.DCVCont.PImin
  Unit Delay{1,3,7..8} (4 alike) : UnitDelay  InitialCondition=[0 0 0]  SampleTime=wt1.Ts_control
  Unit Delay10 : UnitDelay  InitialCondition=1  SampleTime=wt1.Ts_control
  Unit Delay{2,4..5,9} (4 alike) : UnitDelay  SampleTime=wt1.Ts_control
  Unit Delay6 : UnitDelay  InitialCondition=1  SampleTime=wt1.Ts_control
  abc_dq_single_notch_dsc_sfunction : pwrsysTransf/abc_dq_single_notch_dsc_sfunction  Ts=wt1.Ts_control  fn=2*systemBase.fn  zeta=wt1.CurrCont.zeta
  dq_to_abc_single_dual : pwrsysVICtrl/dq_to_abc_single_dual  Ts=wt1.Ts_control  Uabp=wt1.Uabp
  pqui_Transd_NoZeroSeq : pwrsysBasic/pqui_Transd_NoZeroSeq  Sn=wt1.Sn  Uanp=col.Uanp  Iap=wt1.Iap*(wt1.Un/col.Un)
  A : PMIOPort  Port=1  Side=Right
  B : PMIOPort  Port=2  Side=Right
  C : PMIOPort  Port=3  Side=Right
  m : Outport
  wires:
  Divide1/1 -> Enable WT/2  "WT_Idcref_pu"
  Bus Selector/1 -> Unit Delay1/1  "<LV_Vabc>"
  [idq_pos] -> Selector2/1
  Unit Delay2/1 -> Controlled Current Source1/1
  Gain1/1 -> Bus Creator/8, [iabc]  "Iabc_LV_pu"
  Bus Selector/2 -> Unit Delay3/1  "<LV_Iabc>"
  Gain5/1 -> Add1/2
  Math Function/1 -> Add1/1
  Constant6/1 -> Uac_Controller/7, Uac_Controller/6, Uac_Controller/3, Uac_Controller/4
  Constant5/1 -> Enable WT/1
  Add1/1 -> Uac_Controller/2  "vac_drooped"
  Vsp/1 -> Unit Delay10/1
  [mPowerSection] -> Bus Selector/1
  Enable WT/1 -> Unit Delay2/1  "WT_Idcref_pu"
  Gain/1 -> Bus Creator/7, [vabc]  "Vabc_LV_pu"
  Constant2/1 -> Uac_Controller/5
  Constant8/1 -> Udc_Controller/4, Udc_Controller/5
  NotEqual/1 -> Unit Delay5/1
  [vdc] -> Udc_Controller/1
  Unit Delay5/1 -> Udc_Controller/2
  Saturation1/1 -> NotEqual/2, Mux/1  "idref"
  [idc] -> Add/2
  Udc_Controller/1 -> Add/1
  Add/1 -> NotEqual/1, Saturation1/1
  Step/1 -> Udc_Controller/3
  [idq] -> Idq_Dec_Signs_Fdbk_Ref/3
  [Vdc] -> dq_to_abc_single_dual/6
  [wpu] -> Idq_Dec_Signs_Fdbk_Ref/4
  dq_to_abc_single_dual/1 -> DCL_LSC_LCL_Trafo_NoSwitching/2
  Mux/1 -> Idq_Dec_Signs_Fdbk_Ref/1
  Constant3/1 -> DCL_LSC_LCL_Trafo_NoSwitching/1
  Saturation2/1 -> Divide1/2
  Psp/1 -> Unit Delay9/1  "WT_pref"
  [vdc] -> Saturation2/1
  [wt] -> dq_to_abc_single_dual/7
  Constant10/1 -> abc_dq_single_notch_dsc_sfunction/5
  Bus Selector/5 -> Unit Delay7/1  "<HV_Vabc>"
  Bus Selector/6 -> Unit Delay8/1  "<HV_Iabc>"
  pqui_Transd_NoZeroSeq/1 -> Bus Creator/1  "Pavg_pu"
  pqui_Transd_NoZeroSeq/2 -> Bus Creator/2  "Qavg_pu"
  pqui_Transd_NoZeroSeq/3 -> Bus Creator/3  "Vavg_pu"
  pqui_Transd_NoZeroSeq/4 -> Bus Creator/4  "Iavg_pu"
  Bus Creator/1 -> m/1
  Bus Selector/3 -> Unit Delay6/1  "<INV_Vdc>"
  Gain2/1 -> Digital first order LPF4/1, Bus Creator/5  "Vdc_pu"
  Gain4/1 -> [idc], Bus Creator/6  "Idc_pu"
  Bus Selector/4 -> Unit Delay4/1  "<INV_Idc>"
  PLL_pu3/2 -> [wpu]
  PLL_pu3/1 -> [wt]
  Uac_Controller/1 -> Mux/2  "iqref"
  DCL_LSC_LCL_Trafo_NoSwitching/1 -> [mPowerSection]
  Unit Delay1/1 -> Gain/1
  Unit Delay3/1 -> Gain1/1
  Unit Delay4/1 -> Gain4/1
  Unit Delay8/1 -> pqui_Transd_NoZeroSeq/2
  Unit Delay6/1 -> [Vdc], Gain2/1
  Unit Delay7/1 -> pqui_Transd_NoZeroSeq/1
  Unit Delay9/1 -> Divide1/1
  Unit Delay10/1 -> Uac_Controller/1
  abc_dq_single_notch_dsc_sfunction/6 -> Terminator3/1
  abc_dq_single_notch_dsc_sfunction/5 -> Terminator2/1
  Selector2/1 -> Gain5/1
  Idq_Dec_Signs_Fdbk_Ref/2 -> Terminator4/1
  [vdq] -> Idq_Dec_Signs_Fdbk_Ref/2
  Constant1/1 -> dq_to_abc_single_dual/2
  Constant7/1 -> dq_to_abc_single_dual/5
  Constant9/1 -> dq_to_abc_single_dual/4, dq_to_abc_single_dual/3
  Constant11/1 -> Idq_Dec_Signs_Fdbk_Ref/7, Idq_Dec_Signs_Fdbk_Ref/5
  Constant12/1 -> Idq_Dec_Signs_Fdbk_Ref/8, Idq_Dec_Signs_Fdbk_Ref/9, Idq_Dec_Signs_Fdbk_Ref/10, Idq_Dec_Signs_Fdbk_Ref/6
  Idq_Dec_Signs_Fdbk_Ref/3 -> Terminator5/1
  Idq_Dec_Signs_Fdbk_Ref/4 -> [IdqCtrl]
  [IdqCtrl] -> Bus Creator/9
  Idq_Dec_Signs_Fdbk_Ref/1 -> dq_to_abc_single_dual/1
  [wt] -> abc_dq_single_notch_dsc_sfunction/3
  [wpu] -> abc_dq_single_notch_dsc_sfunction/4
  abc_dq_single_notch_dsc_sfunction/1 -> Digital first order LPF2/1
  [vabc] -> abc_dq_single_notch_dsc_sfunction/1, PLL_pu3/1
  [iabc] -> abc_dq_single_notch_dsc_sfunction/2
  abc_dq_single_notch_dsc_sfunction/3 -> Digital first order LPF1/1
  abc_dq_single_notch_dsc_sfunction/4 -> Digital first order LPF/1
  abc_dq_single_notch_dsc_sfunction/2 -> Digital first order LPF3/1
  Digital first order LPF/1 -> [idq_pos]
  Digital first order LPF1/1 -> [vdq_pos]
  [vdq_pos] -> Demux/1
  Demux/1 -> Math Function/1
  Demux/2 -> Math Function/2
  Digital first order LPF2/1 -> [vdq]
  Digital first order LPF3/1 -> [idq]
  Digital first order LPF4/1 -> [vdc]
  connections:
  Controlled Current Source1/RConn1 -- DCL_LSC_LCL_Trafo_NoSwitching/LConn1
  DCL_LSC_LCL_Trafo_NoSwitching/RConn3 -- C/RConn1
  DCL_LSC_LCL_Trafo_NoSwitching/RConn1 -- A/RConn1
  DCL_LSC_LCL_Trafo_NoSwitching/RConn2 -- B/RConn1
  Controlled Current Source1/LConn1 -- DCL_LSC_LCL_Trafo_NoSwitching/LConn2
